simulink model "simulation"  (R2017a)
settings: Solver=VariableStepAuto  StartTime=0.0  StopTime=60000  RelTol=1e-3  EnableMultiTasking=on
settings Model: Creator=DongHe  LastModifiedBy=Administrator
settings OptimizationCC: LifeSpan=inf
settings DebuggingCC: SFUnexpectedBacktrackingDiag=warning  SFNoUnconditionalDefaultTransitionDiag=warning  SFExecutionAtInitializationDiag=none
settings GRTTargetCC: TargetLangStandard=C89/C90 (ANSI)  GeneratePreprocessorConditionals=Disable all
settings ConfigComp: CovMetricSettings=dw  CovHtmlReporting=on  CovSaveCumulativeToWorkspaceVar=on  CovSaveSingleToWorkspaceVar=on  CovExternalEMLEnable=off

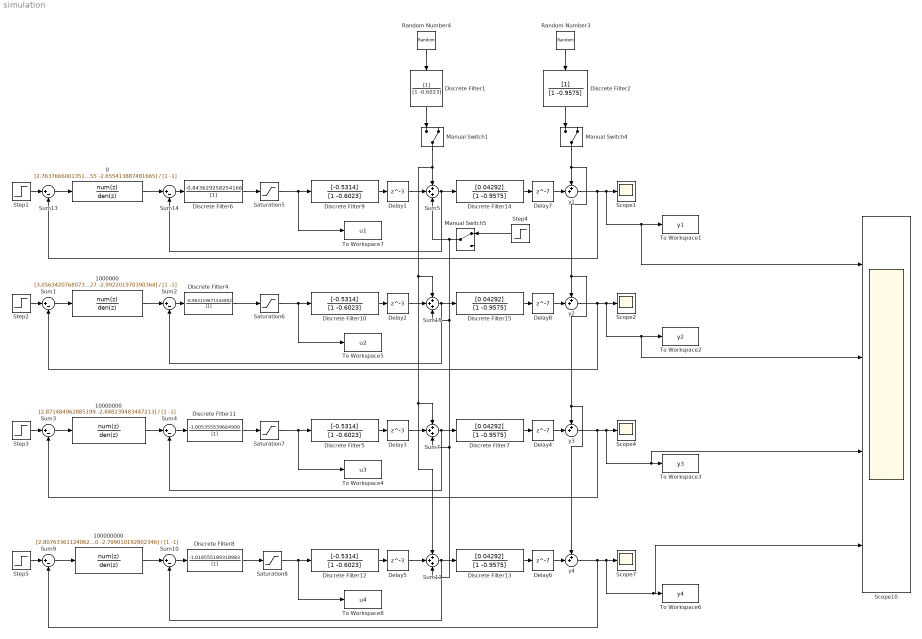
== system simulation ==
  0 : DiscreteFilter  Numerator=[2.763766600135155 -2.655413887481665]  Denominator=[1 -1]  SampleTime=1
  1000000 : DiscreteFilter  Numerator=[3.056342076807327 -2.992201970390364]  Denominator=[1 -1]  SampleTime=1
  10000000 : DiscreteFilter  Numerator=[2.871484962885199 -2.848239483447213]  Denominator=[1 -1]  SampleTime=1
  100000000 : DiscreteFilter  Numerator=[2.807633611240620 -2.799010192802346]  Denominator=[1 -1]  SampleTime=1
  Delay{1..3,5} (4 alike) : Delay  DelayLength=3  SampleTime=1
  Delay{4,6..8} (4 alike) : Delay  DelayLength=7  SampleTime=1
  Discrete Filter1 : DiscreteFilter  Denominator=[1 -0.6023]  SampleTime=1
  Discrete Filter{5,9..10,12} (4 alike) : DiscreteFilter  Numerator=[-0.5314]  Denominator=[1 -0.6023]  SampleTime=1
  Discrete Filter11 : DiscreteFilter  Numerator=-1.005355539664900  Denominator=[1]  SampleTime=1
  Discrete Filter{7,13..15} (4 alike) : DiscreteFilter  Numerator=[0.04292]  Denominator=[1 -0.9575]  SampleTime=1
  Discrete Filter2 : DiscreteFilter  Denominator=[1 -0.9575]  SampleTime=1
  Discrete Filter4 : DiscreteFilter  Numerator=-0.963119671544802  Denominator=[1]  SampleTime=1
  Discrete Filter6 : DiscreteFilter  Numerator=-0.843629258254166  Denominator=[1]  SampleTime=1
  Discrete Filter8 : DiscreteFilter  Numerator=-1.018555189318983  Denominator=[1]  SampleTime=1
  Manual Switch1 : ManualSwitch  CurrentSetting=0
  Manual Switch4 : ManualSwitch  CurrentSetting=0
  Manual Switch5 : ManualSwitch
  Random Number3 : RandomNumber  Variance=0.00005  SampleTime=1
  Random Number4 : RandomNumber  Variance=0.0005  SampleTime=1
  Saturation{5..8} (4 alike) : Saturate  UpperLimit=0  LowerLimit=-16
  Scope{1..2,4,7} (4 alike) : Scope
  Scope10 : Scope  NumInputPorts=4
  Step{1..3,5} (4 alike) : Step  Time=0  After=2  SampleTime=1
  Step4 : Step  Time=30000  After=0.5  SampleTime=1
  Sum{1..4,9..10,13..14} (8 alike) : Sum  Inputs=|+-
  Sum{5,7,11,15} (4 alike) : Sum  Inputs=+++
  To Workspace1 : ToWorkspace  VariableName=y1  SaveFormat=Timeseries  SampleTime=1
  To Workspace2 : ToWorkspace  VariableName=y2  SaveFormat=Timeseries  SampleTime=1
  To Workspace3 : ToWorkspace  VariableName=y3  SaveFormat=Timeseries  SampleTime=1
  To Workspace4 : ToWorkspace  VariableName=u3  SaveFormat=Timeseries  SampleTime=1
  To Workspace5 : ToWorkspace  VariableName=u2  SaveFormat=Timeseries  SampleTime=1
  To Workspace6 : ToWorkspace  VariableName=y4  SaveFormat=Timeseries  SampleTime=1
  To Workspace7 : ToWorkspace  VariableName=u1  SaveFormat=Timeseries  SampleTime=1
  To Workspace8 : ToWorkspace  VariableName=u4  SaveFormat=Timeseries  SampleTime=1
  y{1..4} (4 alike) : Sum  Inputs=++|
  wires:
  Step1/1 -> Sum13/1
  Sum13/1 -> 0/1
  Discrete Filter6/1 -> Saturation5/1
  Sum14/1 -> Discrete Filter6/1
  0/1 -> Sum14/1
  Delay1/1 -> Sum5/2
  Sum5/1 -> Discrete Filter14/1, Sum14/2
  Delay7/1 -> y1/2
  y1/1 -> Scope10/1, To Workspace1/1, Scope1/1, Sum13/2
  Step2/1 -> Sum1/1
  Sum1/1 -> 1000000/1
  Discrete Filter4/1 -> Saturation6/1
  Sum2/1 -> Discrete Filter4/1
  1000000/1 -> Sum2/1
  Delay2/1 -> Sum15/2
  Sum15/1 -> Discrete Filter15/1, Sum2/2
  Delay8/1 -> y2/2
  Random Number4/1 -> Discrete Filter1/1
  Random Number3/1 -> Discrete Filter2/1
  Discrete Filter1/1 -> Manual Switch1/1
  Discrete Filter2/1 -> Manual Switch4/1
  Step4/1 -> Manual Switch5/1
  Discrete Filter9/1 -> Delay1/1
  Discrete Filter10/1 -> Delay2/1
  Discrete Filter14/1 -> Delay7/1
  Discrete Filter15/1 -> Delay8/1
  Saturation5/1 -> Discrete Filter9/1, To Workspace7/1
  Step3/1 -> Sum3/1
  Sum3/1 -> 10000000/1
  Discrete Filter11/1 -> Saturation7/1
  Sum4/1 -> Discrete Filter11/1
  10000000/1 -> Sum4/1
  Delay3/1 -> Sum7/2
  Sum7/1 -> Discrete Filter7/1, Sum4/2
  Delay4/1 -> y3/2
  Discrete Filter5/1 -> Delay3/1
  Discrete Filter7/1 -> Delay4/1
  Step5/1 -> Sum9/1
  Sum9/1 -> 100000000/1
  Discrete Filter8/1 -> Saturation8/1
  Sum10/1 -> Discrete Filter8/1
  100000000/1 -> Sum10/1
  Delay5/1 -> Sum11/2
  Sum11/1 -> Discrete Filter13/1, Sum10/2
  Delay6/1 -> y4/2
  y4/1 -> Scope10/4, To Workspace6/1, Scope7/1, Sum9/2
  Discrete Filter12/1 -> Delay5/1
  Discrete Filter13/1 -> Delay6/1
  Saturation6/1 -> To Workspace5/1, Discrete Filter10/1
  Saturation7/1 -> Discrete Filter5/1, To Workspace4/1
  Saturation8/1 -> Discrete Filter12/1, To Workspace8/1
  Manual Switch1/1 -> Sum11/1, Sum7/1, Sum15/1, Sum5/1
  Manual Switch4/1 -> y4/1, y3/1, y2/1, y1/1
  Manual Switch5/1 -> Sum5/3, Sum11/3, Sum7/3, Sum15/3
  y2/1 -> Scope10/2, To Workspace2/1, Scope2/1, Sum1/2
  y3/1 -> Scope10/3, To Workspace3/1, Scope4/1, Sum3/2
